simulink model "Ejercicio3_modelo"  (R2020a)
settings: Solver=VariableStepAuto  StartTime=0.0  StopTime=60  MaxStep=0.2  RelTol=1e-3
libraries: fl_lib x10, nesl_utility x4
settings Model: Creator=juan  LastModifiedBy=juan

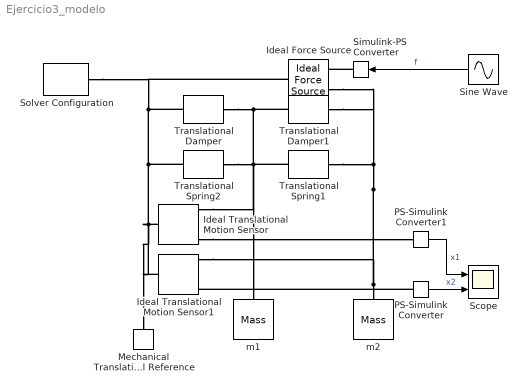
== system Ejercicio3_modelo ==
  Ideal Force Source : fl_lib/Mechanical/Mechanical Sources/Ideal Force Source
  Ideal Translational Motion Sensor : fl_lib/Mechanical/Mechanical Sensors/Ideal Translational Motion Sensor  offset=0 m
  Ideal Translational Motion Sensor1 : fl_lib/Mechanical/Mechanical Sensors/Ideal Translational Motion Sensor  offset=0 m
  Mechanical Translational Reference : fl_lib/Mechanical/Translational Elements/Mechanical Translational Reference
  PS-Simulink Converter : nesl_utility/PS-Simulink Converter  PhysicalDomain=network_engine_domain  SubClassName=ps_output  LeftPortType=input  RightPortType=output  PseudoPeriodic=off  Frequencies=[]  Unit=inherit  AffineConversion=off
  PS-Simulink Converter1 : nesl_utility/PS-Simulink Converter  PhysicalDomain=network_engine_domain  SubClassName=ps_output  LeftPortType=input  RightPortType=output  PseudoPeriodic=off  Frequencies=[]  Unit=inherit  AffineConversion=off
  Scope : Scope  NumInputPorts=2
  Simulink-PS Converter : nesl_utility/Simulink-PS Converter  PhysicalDomain=network_engine_domain  SubClassName=ps_input  LeftPortType=input  RightPortType=output  PseudoPeriodic=off  Frequencies=[]  NoiseDistribution=none  NoiseParameters=[]  Unit=1  AffineConversion=off  FilteringAndDerivatives=provide  SimscapeFilterOrder=1  InputFilterTimeConstant=0.001  UdotUserProvided=0
  Sine Wave : Sin  SampleTime=0
  Solver Configuration : nesl_utility/Solver Configuration  PhysicalDomain=network_engine_domain  SubClassName=solver  LeftPortType=input  RightPortType=generic  Tones=[]  Harmonics=[]  SimulateNoise=off  Profile=off  UseLocalSampling=off  EnableSwitchedLinearOptims=on  FrequencyDomain=off  UseCCode=off  RelTol=0.001  AbsTol=1e-06  MinStep=1e-09  ToWorkspace=off  RevertToSquareIcSolve=off  NumHomotopyIterations=100  PhasorMode=off  PhasorModeNumHarmonics=1  DoDC=off  ResidualTolerance=1e-09  UseLocalSolver=off  LocalSolverChoice=NE_BACKWARD_EULER_ADVANCER  LocalSolverSampleTime=0.001  DoFixedCost=off  MaxNonlinIter=3  MaxModeIter=2  LinearAlgebra=auto  EquationFormulation=NE_TIME_EF  DelaysMemoryBudget=1024  AutomaticFiltering=on  FilteringTimeConstant=0.001  PartitionStorageMethod=AS_NEEDED  PartitionMemoryBudget=1024  PartitionMethod=ROBUST
  Translational Damper : fl_lib/Mechanical/Translational Elements/Translational Damper  D=50 N/(m/s)  v_specify=off  v_priority=None  v=0 m/s  v_nominal_specify=off  v_nominal_unit=m/s  v_nominal_value=1  f_specify=off  f_priority=None  f=0 N  f_nominal_specify=off  f_nominal_unit=N  f_nominal_value=1
      settings: AttributesFormatString=|
      | %<D>
      | %<D_unit>
  Translational Damper1 : fl_lib/Mechanical/Translational Elements/Translational Damper  D=50 N/(m/s)  v_specify=off  v_priority=None  v=0 m/s  v_nominal_specify=off  v_nominal_unit=m/s  v_nominal_value=1  f_specify=off  f_priority=None  f=0 N  f_nominal_specify=off  f_nominal_unit=N  f_nominal_value=1
      settings: AttributesFormatString=|
      | %<D>
      | %<D_unit>
  Translational Spring1 : fl_lib/Mechanical/Translational Elements/Translational Spring  spr_rate=104*1.5 N/m  v_specify=off  v_priority=None  v=0 m/s  v_nominal_specify=off  v_nominal_unit=m/s  v_nominal_value=1  f_specify=off  f_priority=None  f=0 N  f_nominal_specify=off  f_nominal_unit=N  f_nominal_value=1  x_specify=off  x_priority=High  x=0 m  x_nominal_specify=off  x_nominal_unit=m  x_nominal_value=1
      settings: AttributesFormatString=|
      | %<spr_rate>
      | %<spr_rate_unit>
  Translational Spring2 : fl_lib/Mechanical/Translational Elements/Translational Spring  spr_rate=104 N/m  v_specify=off  v_priority=None  v=0 m/s  v_nominal_specify=off  v_nominal_unit=m/s  v_nominal_value=1  f_specify=off  f_priority=None  f=0 N  f_nominal_specify=off  f_nominal_unit=N  f_nominal_value=1  x_specify=off  x_priority=High  x=0 m  x_nominal_specify=off  x_nominal_unit=m  x_nominal_value=1
      settings: AttributesFormatString=|
      | %<spr_rate>
      | %<spr_rate_unit>
  m1 : fl_lib/Mechanical/Translational Elements/Mass  mass=50 kg  v_specify=off  v_priority=High  v=0 m/s  v_nominal_specify=off  v_nominal_unit=m/s  v_nominal_value=1  f_specify=off  f_priority=None  f=0 N  f_nominal_specify=off  f_nominal_unit=N  f_nominal_value=1
      settings: AttributesFormatString=|
      | %<mass>
      | %<mass_unit>
  m2 : fl_lib/Mechanical/Translational Elements/Mass  mass=50 kg  v_specify=off  v_priority=High  v=0 m/s  v_nominal_specify=off  v_nominal_unit=m/s  v_nominal_value=1  f_specify=off  f_priority=None  f=0 N  f_nominal_specify=off  f_nominal_unit=N  f_nominal_value=1
      settings: AttributesFormatString=|
      | %<mass>
      | %<mass_unit>
  wires:
  Sine Wave/1 -> Simulink-PS Converter/1  "f"
  PS-Simulink Converter1/1 -> Scope/1  "x1"
  PS-Simulink Converter/1 -> Scope/2  "x2"
  connections:
  Translational Damper/LConn1 -- Mechanical Translational Reference/LConn1 -- Ideal Translational Motion Sensor1/LConn1 -- Ideal Translational Motion Sensor/LConn1 -- Translational Spring2/LConn1 -- Solver Configuration/RConn1 -- Ideal Force Source/LConn1
  Translational Damper/RConn1 -- Translational Damper1/LConn1 -- Translational Spring1/LConn1 -- Ideal Translational Motion Sensor/RConn1 -- m1/LConn1 -- Translational Spring2/RConn1
  m2/LConn1 -- Translational Damper1/RConn1 -- Ideal Force Source/RConn2 -- Translational Spring1/RConn1 -- Ideal Translational Motion Sensor1/RConn1
  Simulink-PS Converter/RConn1 -- Ideal Force Source/RConn1
  Ideal Translational Motion Sensor/RConn3 -- PS-Simulink Converter1/LConn1
  PS-Simulink Converter/LConn1 -- Ideal Translational Motion Sensor1/RConn3
